simulink subsystem "Catmull_Rom_Combine"  (R2023b)
settings: Solver=VariableStepAuto  StartTime=0.0  StopTime=10.0  RelTol=1e-3
undefined symbols (not defined in the file): Spline_Tension
settings Model: Creator=FIRSTMentor  LastModifiedBy=FIRSTMentor

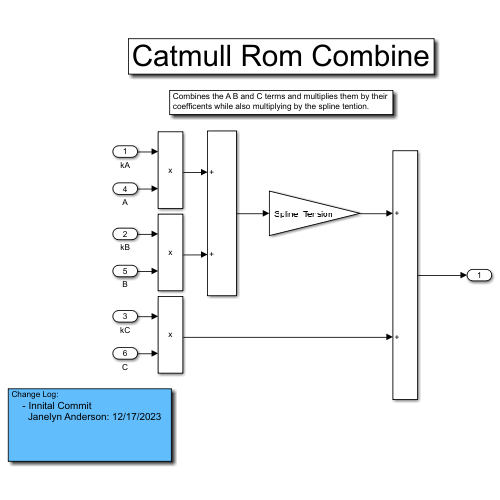
[thumbnail: Simulink's stored preview of the top-level diagram]
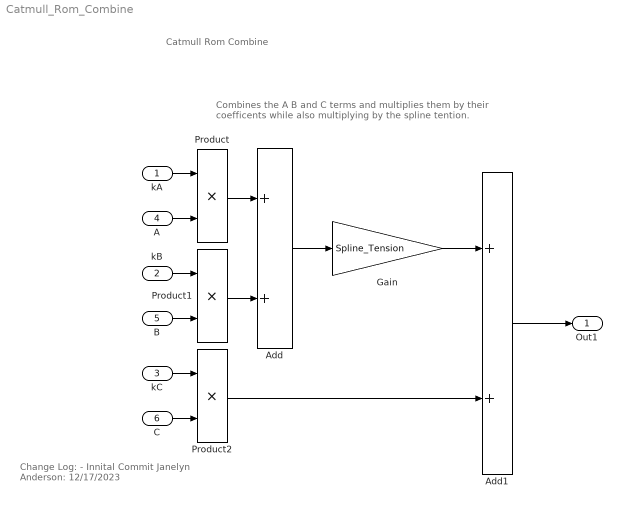
== system Catmull_Rom_Combine ==
  note: Catmull Rom Combine
  note: Combines the A B and C terms and multiplies them by their coefficents while also multiplying by the spline tention.
  note: Change Log:
      | - Innital Commit
      | Janelyn Anderson: 12/17/2023
  kA : Inport
  kB : Inport  Port=2
  kC : Inport  Port=3
  A : Inport  Port=4
  B : Inport  Port=5
  C : Inport  Port=6
  Add : Sum  Inputs=2
  Add1 : Sum
  Gain : Gain  Gain=Spline_Tension
  Product : Product
  Product1 : Product
  Product2 : Product
  Out1 : Outport
  wires:
  Gain/1 -> Add1/1
  Add1/1 -> Out1/1
  kA/1 -> Product/1
  Product1/1 -> Add/2
  C/1 -> Product2/2
  kC/1 -> Product2/1
  A/1 -> Product/2
  Add/1 -> Gain/1
  Product2/1 -> Add1/2
  Product/1 -> Add/1
  kB/1 -> Product1/1
  B/1 -> Product1/2
